simulink model "simulate_motorR2011a"  (Simulink 7.7)
settings: Solver=ode45  StartTime=0.0  StopTime=5  FixedStep=0.001  RelTol=1e-3
values from neighbouring files (symbols this model uses):
  L = 0.8    [cart_and_pendulum.m]
undefined symbols (not defined in the file or in its folder): Bm, Jm, Kb, Km, R
settings Model: Creator=arturo  LastModifiedBy=arturogilaparicio
settings DataIOCC: LimitDataPoints=off
settings CodeAppCC: CustomSymbolStrType=$N$R$M_T
settings GRTTargetCC: TargetFunctionLibrary=C89/C90 (ANSI)

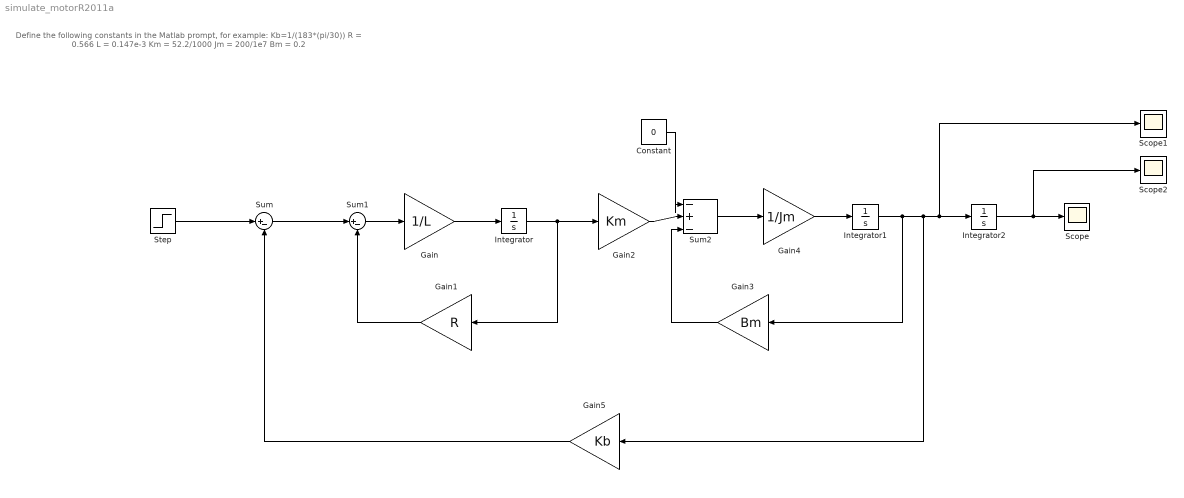
== system simulate_motorR2011a ==
  note: Define the following constants in the Matlab prompt, for example:
      | Kb=1/(183*(pi/30))
      | R = 0.566
      | L = 0.147e-3
      | Km = 52.2/1000
      | Jm = 200/1e7
      | Bm = 0.2
  Constant : Constant  Value=0
  Gain : Gain  Gain=1/L
  Gain1 : Gain  Gain=R
  Gain2 : Gain  Gain=Km
  Gain3 : Gain  Gain=Bm
  Gain4 : Gain  Gain=1/Jm
  Gain5 : Gain  Gain=Kb
  Integrator : Integrator
  Integrator1 : Integrator
  Integrator2 : Integrator
  Scope : Scope
  Scope1 : Scope
  Scope2 : Scope
      settings: SaveName=ScopeData2
  Step : Step  Time=0  After=5  SampleTime=0
  Sum : Sum  Inputs=|+-
  Sum1 : Sum  Inputs=|+-
  Sum2 : Sum  Inputs=|-+-
  wires:
  Step/1 -> Sum/1
  Sum/1 -> Sum1/1
  Sum1/1 -> Gain/1
  Gain/1 -> Integrator/1
  Gain1/1 -> Sum1/2
  Integrator/1 -> Gain2/1, Gain1/1
  Constant/1 -> Sum2/1
  Gain2/1 -> Sum2/2
  Gain3/1 -> Sum2/3
  Gain4/1 -> Integrator1/1
  Sum2/1 -> Gain4/1
  Integrator1/1 -> Scope1/1, Integrator2/1, Gain5/1, Gain3/1
  Gain5/1 -> Sum/2
  Integrator2/1 -> Scope2/1, Scope/1
